simulink model "simscape_special_switch_1"  (R2022b)
settings: Solver=VariableStepAuto  StartTime=0.0  StopTime=10.0  RelTol=1e-3
libraries: spsDiodeLib x1, spsIdealSwitchLib x1
settings Model: Creator=Hyeongmeen Baik  LastModifiedBy=Hyeongmeen Baik

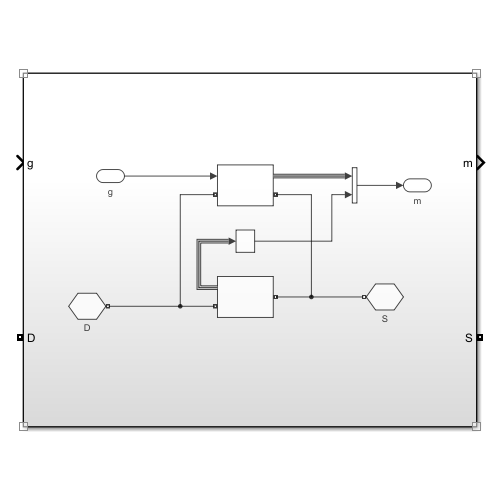
[thumbnail: Simulink's stored preview of the top-level diagram]
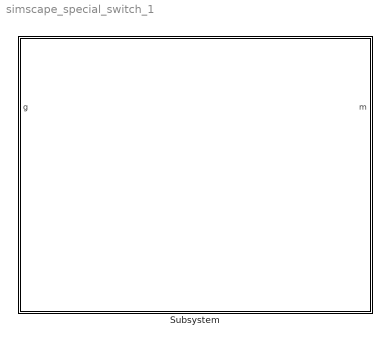
== system simscape_special_switch_1 ==
  Subsystem : Subsystem

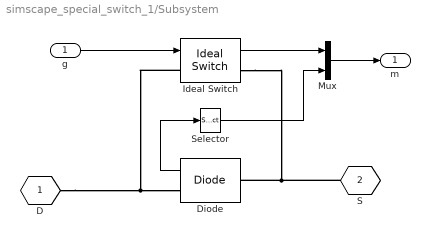
== system simscape_special_switch_1/Subsystem ==
  g : Inport
  Diode : spsDiodeLib/Diode  Ron=1e-3  Lon=0  Vf=Vf  IC=0  UseSnubber=0  Rs=inf  Cs=0  Measurements=on
  Ideal Switch : spsIdealSwitchLib/Ideal Switch  Ron=1e-3  Lon=0  IC=0  Rs=Rs_fet  Cs=Cs_fet  Measurements=on
  Mux : Mux  Inputs=[2,1]
  Selector : Selector  InputPortWidth=2  IndexOptions=Index vector (dialog)  Indices=1  OutputSizes=1
  D : PMIOPort  Tag=PMCPort  Side=Left
  S : PMIOPort  Tag=PMCPort  Port=2  Side=Right
  m : Outport  VectorParamsAs1DForOutWhenUnconnected=off
  wires:
  Ideal Switch/1 -> Mux/1
  Diode/1 -> Selector/1
  Mux/1 -> m/1
  g/1 -> Ideal Switch/1
  Selector/1 -> Mux/2
  connections:
  Ideal Switch/LConn1 -- Diode/RConn1 -- D/RConn1
  Ideal Switch/RConn1 -- Diode/LConn1 -- S/RConn1
